simulink model "Ycap_snt"  (R2025b)
settings: Solver=ode45  StartTime=0.0  StopTime=10.0  RelTol=1e-3  EnableMultiTasking=on
undefined symbols (not defined in the file or in its folder): DiscIntNeverNeededParam, Ts
libraries: fl_lib x24, nesl_utility x12
(part 3 of 3)

== system Ycap_snt/3sscT/constPQ2/single-phase PQ/Vectorized PQ meas ==
  V : Inport
  I : Inport  Port=2
  Product1 : Product  InputSameDT=on  SaturateOnIntegerOverflow=on  OutDataTypeStr=Inherit: Same as first input
  Product3 : Product  InputSameDT=on  SaturateOnIntegerOverflow=on  OutDataTypeStr=Inherit: Same as first input
  Sum1 : Sum  Inputs=1  CollapseMode=Specified dimension  InputSameDT=on  SaturateOnIntegerOverflow=on  OutDataTypeStr=Inherit: Same as first input
  Sum2 : Sum  Inputs=1  CollapseMode=Specified dimension  InputSameDT=on  SaturateOnIntegerOverflow=on  OutDataTypeStr=Inherit: Same as first input
  Sum4 : Sum  Inputs=+-  InputSameDT=on  SaturateOnIntegerOverflow=on  OutDataTypeStr=Inherit: Same as first input
  pu->V : Gain  Gain=1/sqrt(3)  SaturateOnIntegerOverflow=on  OutDataTypeStr=Inherit: Same as input  ParamDataTypeStr=Inherit: Same as input
  pu->V1 : Gain  Gain=[0 1 0;0 0 1;1 0 0]  Multiplication=Matrix(K*u)  SaturateOnIntegerOverflow=on  OutDataTypeStr=Inherit: Same as input  ParamDataTypeStr=Inherit: Same as input
  pu->V2 : Gain  Gain=[0 1 0;0 0 1;1 0 0]  Multiplication=Matrix(K*u)  SaturateOnIntegerOverflow=on  OutDataTypeStr=Inherit: Same as input  ParamDataTypeStr=Inherit: Same as input
  P : Outport  VectorParamsAs1DForOutWhenUnconnected=off
  Q : Outport  Port=2  VectorParamsAs1DForOutWhenUnconnected=off
  wires:
  pu->V2/1 -> Product3/1
  Sum4/1 -> pu->V2/1  "VV2"
  pu->V1/1 -> Sum4/2
  Sum2/1 -> P/1
  I/1 -> Product1/2, Product3/2
  V/1 -> Product1/1, pu->V1/1, Sum4/1  "VV1"
  Product1/1 -> Sum2/1
  Product3/1 -> Sum1/1
  Sum1/1 -> pu->V/1
  pu->V/1 -> Q/1

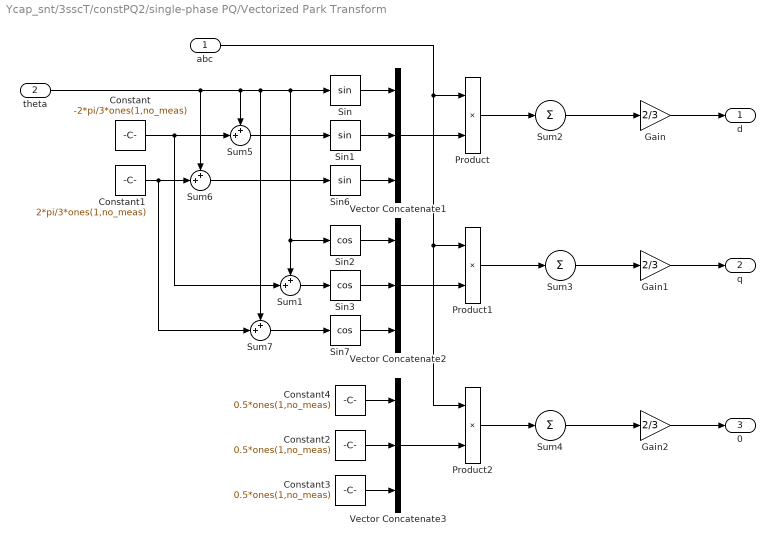
== system Ycap_snt/3sscT/constPQ2/single-phase PQ/Vectorized Park Transform ==
  abc : Inport
  theta : Inport  Port=2
  Constant : Constant  Value=-2*pi/3*ones(1,no_meas)  VectorParams1D=off  SampleTime=Ts
  Constant1 : Constant  Value=2*pi/3*ones(1,no_meas)  VectorParams1D=off  SampleTime=Ts
  Constant2 : Constant  Value=0.5*ones(1,no_meas)  VectorParams1D=off  SampleTime=Ts
  Constant3 : Constant  Value=0.5*ones(1,no_meas)  VectorParams1D=off  SampleTime=Ts
  Constant4 : Constant  Value=0.5*ones(1,no_meas)  VectorParams1D=off  SampleTime=Ts
  Gain : Gain  Gain=2/3
  Gain1 : Gain  Gain=2/3
  Gain2 : Gain  Gain=2/3
  Product : Product
  Product1 : Product
  Product2 : Product
  Sin : Trigonometry
  Sin1 : Trigonometry
  Sin2 : Trigonometry  Operator=cos
  Sin3 : Trigonometry  Operator=cos
  Sin6 : Trigonometry
  Sin7 : Trigonometry  Operator=cos
  Sum{1,5..7} (4 alike) : Sum  Inputs=++|
  Sum2 : Sum  Inputs=1  CollapseMode=Specified dimension  InputSameDT=on  SaturateOnIntegerOverflow=on  OutDataTypeStr=Inherit: Same as first input
  Sum3 : Sum  Inputs=1  CollapseMode=Specified dimension  InputSameDT=on  SaturateOnIntegerOverflow=on  OutDataTypeStr=Inherit: Same as first input
  Sum4 : Sum  Inputs=1  CollapseMode=Specified dimension  InputSameDT=on  SaturateOnIntegerOverflow=on  OutDataTypeStr=Inherit: Same as first input
  Vector Concatenate1 : Concatenate  NumInputs=3  Mode=Multidimensional array
  Vector Concatenate2 : Concatenate  NumInputs=3  Mode=Multidimensional array
  Vector Concatenate3 : Concatenate  NumInputs=3  Mode=Multidimensional array
  d : Outport  VectorParamsAs1DForOutWhenUnconnected=off
  q : Outport  Port=2  VectorParamsAs1DForOutWhenUnconnected=off
  0 : Outport  Port=3  VectorParamsAs1DForOutWhenUnconnected=off
  wires:
  theta/1 -> Sum7/1, Sin/1, Sum1/1, Sin2/1, Sum5/1, Sum6/1
  Sum7/1 -> Sin7/1
  Sum1/1 -> Sin3/1
  Constant1/1 -> Sum6/2, Sum7/2
  Constant/1 -> Sum5/2, Sum1/2
  Sum6/1 -> Sin6/1
  Sum5/1 -> Sin1/1
  abc/1 -> Product2/1, Product1/1, Product/1
  Sin/1 -> Vector Concatenate1/1
  Sin1/1 -> Vector Concatenate1/2
  Sin3/1 -> Vector Concatenate2/2
  Sin2/1 -> Vector Concatenate2/1
  Constant4/1 -> Vector Concatenate3/1
  Constant2/1 -> Vector Concatenate3/2
  Sin6/1 -> Vector Concatenate1/3
  Sin7/1 -> Vector Concatenate2/3
  Constant3/1 -> Vector Concatenate3/3
  Vector Concatenate3/1 -> Product2/2
  Vector Concatenate2/1 -> Product1/2
  Vector Concatenate1/1 -> Product/2
  Product/1 -> Sum2/1
  Product1/1 -> Sum3/1
  Product2/1 -> Sum4/1
  Sum3/1 -> Gain1/1
  Sum4/1 -> Gain2/1
  Sum2/1 -> Gain/1
  Gain2/1 -> 0/1
  Gain1/1 -> q/1
  Gain/1 -> d/1

== system Ycap_snt/3sscT/constPQ2/single-phase PQ/Vectorized Inverse Clarke Transform ==
  alphabeta0 : Inport
  Constant1 : Constant  Value=zeros(1,no_meas)  VectorParams1D=off  SampleTime=Ts
  Constant2 : Constant  Value=sqrt(3)/2*ones(1,no_meas)  VectorParams1D=off  SampleTime=Ts
  Constant3 : Constant  Value=sqrt(1/2)*ones(1,no_meas)  VectorParams1D=off  SampleTime=Ts
  Constant4 : Constant  Value=-0.5*ones(1,no_meas)  VectorParams1D=off  SampleTime=Ts
  Constant5 : Constant  Value=sqrt(1/2)*ones(1,no_meas)  VectorParams1D=off  SampleTime=Ts
  Constant6 : Constant  Value=ones(1,no_meas)  VectorParams1D=off  SampleTime=Ts
  Constant7 : Constant  Value=-sqrt(3)/2*ones(1,no_meas)  VectorParams1D=off  SampleTime=Ts
  Constant8 : Constant  Value=sqrt(1/2)*ones(1,no_meas)  VectorParams1D=off  SampleTime=Ts
  Constant9 : Constant  Value=-0.5*ones(1,no_meas)  VectorParams1D=off  SampleTime=Ts
  Gain : Gain  Gain=sqrt(2/3)
  Gain1 : Gain  Gain=sqrt(2/3)
  Gain2 : Gain  Gain=sqrt(2/3)
  Product : Product
  Product1 : Product
  Product2 : Product
  Sum2 : Sum  Inputs=1  CollapseMode=Specified dimension  InputSameDT=on  SaturateOnIntegerOverflow=on  OutDataTypeStr=Inherit: Same as first input
  Sum3 : Sum  Inputs=1  CollapseMode=Specified dimension  InputSameDT=on  SaturateOnIntegerOverflow=on  OutDataTypeStr=Inherit: Same as first input
  Sum4 : Sum  Inputs=1  CollapseMode=Specified dimension  InputSameDT=on  SaturateOnIntegerOverflow=on  OutDataTypeStr=Inherit: Same as first input
  Vector Concatenate1 : Concatenate  NumInputs=3  Mode=Multidimensional array
  Vector Concatenate2 : Concatenate  NumInputs=3  Mode=Multidimensional array
  Vector Concatenate3 : Concatenate  NumInputs=3  Mode=Multidimensional array
  a : Outport  VectorParamsAs1DForOutWhenUnconnected=off
  b : Outport  Port=2  VectorParamsAs1DForOutWhenUnconnected=off
  c : Outport  Port=3  VectorParamsAs1DForOutWhenUnconnected=off
  wires:
  Constant8/1 -> Vector Concatenate3/3
  Constant7/1 -> Vector Concatenate3/2
  Constant9/1 -> Vector Concatenate3/1
  alphabeta0/1 -> Product/1, Product1/1, Product2/1
  Gain2/1 -> c/1
  Gain1/1 -> b/1
  Gain/1 -> a/1
  Product2/1 -> Sum4/1
  Product1/1 -> Sum3/1
  Product/1 -> Sum2/1
  Vector Concatenate1/1 -> Product/2
  Vector Concatenate2/1 -> Product1/2
  Vector Concatenate3/1 -> Product2/2
  Constant3/1 -> Vector Concatenate2/3
  Constant5/1 -> Vector Concatenate1/3
  Constant4/1 -> Vector Concatenate2/1
  Constant2/1 -> Vector Concatenate2/2
  Constant1/1 -> Vector Concatenate1/2
  Constant6/1 -> Vector Concatenate1/1
  Sum2/1 -> Gain/1
  Sum3/1 -> Gain1/1
  Sum4/1 -> Gain2/1

== system Ycap_snt/3sscT/constPQ2/single-phase PQ/Vectorized Inverse Park Transform ==
  dq0 : Inport
  theta : Inport  Port=2
  Constant : Constant  Value=-2*pi/3*ones(1,no_meas)  VectorParams1D=off  SampleTime=Ts
  Constant1 : Constant  Value=2*pi/3*ones(1,no_meas)  VectorParams1D=off  SampleTime=Ts
  Constant2 : Constant  Value=ones(1,no_meas)  VectorParams1D=off  SampleTime=Ts
  Constant3 : Constant  Value=ones(1,no_meas)  VectorParams1D=off  SampleTime=Ts
  Constant4 : Constant  Value=ones(1,no_meas)  VectorParams1D=off  SampleTime=Ts
  Product : Product
  Product1 : Product
  Product2 : Product
  Sin : Trigonometry
  Sin1 : Trigonometry  Operator=cos
  Sin2 : Trigonometry
  Sin3 : Trigonometry  Operator=cos
  Sin4 : Trigonometry
  Sin5 : Trigonometry  Operator=cos
  Sum : Sum  Inputs=++|
  Sum1 : Sum  Inputs=++|
  Sum2 : Sum  Inputs=1  CollapseMode=Specified dimension  InputSameDT=on  SaturateOnIntegerOverflow=on  OutDataTypeStr=Inherit: Same as first input
  Sum3 : Sum  Inputs=1  CollapseMode=Specified dimension  InputSameDT=on  SaturateOnIntegerOverflow=on  OutDataTypeStr=Inherit: Same as first input
  Sum4 : Sum  Inputs=1  CollapseMode=Specified dimension  InputSameDT=on  SaturateOnIntegerOverflow=on  OutDataTypeStr=Inherit: Same as first input
  Vector Concatenate1 : Concatenate  NumInputs=3  Mode=Multidimensional array
  Vector Concatenate2 : Concatenate  NumInputs=3  Mode=Multidimensional array
  Vector Concatenate3 : Concatenate  NumInputs=3  Mode=Multidimensional array
  a : Outport  VectorParamsAs1DForOutWhenUnconnected=off
  b : Outport  Port=2  VectorParamsAs1DForOutWhenUnconnected=off
  c : Outport  Port=3  VectorParamsAs1DForOutWhenUnconnected=off
  wires:
  Product2/1 -> Sum4/1
  Product1/1 -> Sum3/1
  Product/1 -> Sum2/1
  Vector Concatenate1/1 -> Product/2
  Vector Concatenate2/1 -> Product1/2
  Vector Concatenate3/1 -> Product2/2
  Constant3/1 -> Vector Concatenate3/3
  Constant4/1 -> Vector Concatenate2/3
  Constant2/1 -> Vector Concatenate1/3
  Sin5/1 -> Vector Concatenate3/2
  Sin4/1 -> Vector Concatenate3/1
  Sum1/1 -> Sin5/1, Sin4/1
  Constant1/1 -> Sum1/1
  Constant/1 -> Sum/1
  Sum/1 -> Sin2/1, Sin3/1
  Sin2/1 -> Vector Concatenate2/1
  Sin3/1 -> Vector Concatenate2/2
  Sin1/1 -> Vector Concatenate1/2
  Sin/1 -> Vector Concatenate1/1
  dq0/1 -> Product/1, Product1/1, Product2/1
  theta/1 -> Sum/2, Sin/1, Sum1/2, Sin1/1
  Sum2/1 -> a/1
  Sum3/1 -> b/1
  Sum4/1 -> c/1

== system Ycap_snt/3sscT/constPQ3/single-phase PQ/Subsystem ==
  In1 : Inport
  Discrete-Time Integrator : DiscreteIntegrator  gainval=1/Ts/20  InitialCondition=2000  SampleTime=-1  ICPrevOutput=DiscIntNeverNeededParam  ICPrevScaledInput=DiscIntNeverNeededParam
  Sum : Sum  Inputs=|+-
  Out1 : Outport
  wires:
  In1/1 -> Sum/1
  Sum/1 -> Discrete-Time Integrator/1
  Discrete-Time Integrator/1 -> Sum/2, Out1/1

== system Ycap_snt/3sscT/constPQ3/single-phase PQ/Vectorized Clarke Transform ==
  abc : Inport
  Constant1 : Constant  Value=-0.5*ones(1,no_meas)  VectorParams1D=off  SampleTime=Ts
  Constant{2..4,6} (4 alike) : Constant  Value=ones(1,no_meas)  VectorParams1D=off  SampleTime=Ts
  Constant5 : Constant  Value=-0.5*ones(1,no_meas)  VectorParams1D=off  SampleTime=Ts
  Constant7 : Constant  Value=zeros(1,no_meas)  VectorParams1D=off  SampleTime=Ts
  Constant8 : Constant  Value=sqrt(3)/2*ones(1,no_meas)  VectorParams1D=off  SampleTime=Ts
  Constant9 : Constant  Value=-sqrt(3)/2*ones(1,no_meas)  VectorParams1D=off  SampleTime=Ts
  Gain : Gain  Gain=sqrt(2/3)
  Gain1 : Gain  Gain=sqrt(2/3)
  Gain2 : Gain  Gain=sqrt(1/3)
  Product : Product
  Product1 : Product
  Product2 : Product
  Sum2 : Sum  Inputs=1  CollapseMode=Specified dimension  InputSameDT=on  SaturateOnIntegerOverflow=on  OutDataTypeStr=Inherit: Same as first input
  Sum3 : Sum  Inputs=1  CollapseMode=Specified dimension  InputSameDT=on  SaturateOnIntegerOverflow=on  OutDataTypeStr=Inherit: Same as first input
  Sum4 : Sum  Inputs=1  CollapseMode=Specified dimension  InputSameDT=on  SaturateOnIntegerOverflow=on  OutDataTypeStr=Inherit: Same as first input
  Vector Concatenate1 : Concatenate  NumInputs=3  Mode=Multidimensional array
  Vector Concatenate2 : Concatenate  NumInputs=3  Mode=Multidimensional array
  Vector Concatenate3 : Concatenate  NumInputs=3  Mode=Multidimensional array
  alpha : Outport  VectorParamsAs1DForOutWhenUnconnected=off
  beta : Outport  Port=2  VectorParamsAs1DForOutWhenUnconnected=off
  zero : Outport  Port=3  VectorParamsAs1DForOutWhenUnconnected=off
  wires:
  Gain/1 -> alpha/1
  Gain1/1 -> beta/1
  Gain2/1 -> zero/1
  Sum2/1 -> Gain/1
  Sum4/1 -> Gain2/1
  Sum3/1 -> Gain1/1
  Product2/1 -> Sum4/1
  Product1/1 -> Sum3/1
  Product/1 -> Sum2/1
  Vector Concatenate1/1 -> Product/2
  Vector Concatenate2/1 -> Product1/2
  Vector Concatenate3/1 -> Product2/2
  Constant3/1 -> Vector Concatenate3/3
  Constant2/1 -> Vector Concatenate3/2
  Constant4/1 -> Vector Concatenate3/1
  abc/1 -> Product/1, Product1/1, Product2/1
  Constant6/1 -> Vector Concatenate1/1
  Constant1/1 -> Vector Concatenate1/2
  Constant5/1 -> Vector Concatenate1/3
  Constant7/1 -> Vector Concatenate2/1
  Constant8/1 -> Vector Concatenate2/2
  Constant9/1 -> Vector Concatenate2/3

== system Ycap_snt/3sscT/constPQ3/single-phase PQ/Vectorized PQ meas ==
  V : Inport
  I : Inport  Port=2
  Product1 : Product  InputSameDT=on  SaturateOnIntegerOverflow=on  OutDataTypeStr=Inherit: Same as first input
  Product3 : Product  InputSameDT=on  SaturateOnIntegerOverflow=on  OutDataTypeStr=Inherit: Same as first input
  Sum1 : Sum  Inputs=1  CollapseMode=Specified dimension  InputSameDT=on  SaturateOnIntegerOverflow=on  OutDataTypeStr=Inherit: Same as first input
  Sum2 : Sum  Inputs=1  CollapseMode=Specified dimension  InputSameDT=on  SaturateOnIntegerOverflow=on  OutDataTypeStr=Inherit: Same as first input
  Sum4 : Sum  Inputs=+-  InputSameDT=on  SaturateOnIntegerOverflow=on  OutDataTypeStr=Inherit: Same as first input
  pu->V : Gain  Gain=1/sqrt(3)  SaturateOnIntegerOverflow=on  OutDataTypeStr=Inherit: Same as input  ParamDataTypeStr=Inherit: Same as input
  pu->V1 : Gain  Gain=[0 1 0;0 0 1;1 0 0]  Multiplication=Matrix(K*u)  SaturateOnIntegerOverflow=on  OutDataTypeStr=Inherit: Same as input  ParamDataTypeStr=Inherit: Same as input
  pu->V2 : Gain  Gain=[0 1 0;0 0 1;1 0 0]  Multiplication=Matrix(K*u)  SaturateOnIntegerOverflow=on  OutDataTypeStr=Inherit: Same as input  ParamDataTypeStr=Inherit: Same as input
  P : Outport  VectorParamsAs1DForOutWhenUnconnected=off
  Q : Outport  Port=2  VectorParamsAs1DForOutWhenUnconnected=off
  wires:
  pu->V/1 -> Q/1
  Sum1/1 -> pu->V/1
  Product3/1 -> Sum1/1
  Product1/1 -> Sum2/1
  V/1 -> Sum4/1, pu->V1/1, Product1/1  "VV1"
  I/1 -> Product3/2, Product1/2
  Sum2/1 -> P/1
  pu->V1/1 -> Sum4/2
  Sum4/1 -> pu->V2/1  "VV2"
  pu->V2/1 -> Product3/1

== system Ycap_snt/3sscT/constPQ3/single-phase PQ/Vectorized Park Transform ==
  abc : Inport
  theta : Inport  Port=2
  Constant : Constant  Value=-2*pi/3*ones(1,no_meas)  VectorParams1D=off  SampleTime=Ts
  Constant1 : Constant  Value=2*pi/3*ones(1,no_meas)  VectorParams1D=off  SampleTime=Ts
  Constant2 : Constant  Value=0.5*ones(1,no_meas)  VectorParams1D=off  SampleTime=Ts
  Constant3 : Constant  Value=0.5*ones(1,no_meas)  VectorParams1D=off  SampleTime=Ts
  Constant4 : Constant  Value=0.5*ones(1,no_meas)  VectorParams1D=off  SampleTime=Ts
  Gain : Gain  Gain=2/3
  Gain1 : Gain  Gain=2/3
  Gain2 : Gain  Gain=2/3
  Product : Product
  Product1 : Product
  Product2 : Product
  Sin : Trigonometry
  Sin1 : Trigonometry
  Sin2 : Trigonometry  Operator=cos
  Sin3 : Trigonometry  Operator=cos
  Sin6 : Trigonometry
  Sin7 : Trigonometry  Operator=cos
  Sum{1,5..7} (4 alike) : Sum  Inputs=++|
  Sum2 : Sum  Inputs=1  CollapseMode=Specified dimension  InputSameDT=on  SaturateOnIntegerOverflow=on  OutDataTypeStr=Inherit: Same as first input
  Sum3 : Sum  Inputs=1  CollapseMode=Specified dimension  InputSameDT=on  SaturateOnIntegerOverflow=on  OutDataTypeStr=Inherit: Same as first input
  Sum4 : Sum  Inputs=1  CollapseMode=Specified dimension  InputSameDT=on  SaturateOnIntegerOverflow=on  OutDataTypeStr=Inherit: Same as first input
  Vector Concatenate1 : Concatenate  NumInputs=3  Mode=Multidimensional array
  Vector Concatenate2 : Concatenate  NumInputs=3  Mode=Multidimensional array
  Vector Concatenate3 : Concatenate  NumInputs=3  Mode=Multidimensional array
  d : Outport  VectorParamsAs1DForOutWhenUnconnected=off
  q : Outport  Port=2  VectorParamsAs1DForOutWhenUnconnected=off
  0 : Outport  Port=3  VectorParamsAs1DForOutWhenUnconnected=off
  wires:
  Gain/1 -> d/1
  Gain1/1 -> q/1
  Gain2/1 -> 0/1
  Sum2/1 -> Gain/1
  Sum4/1 -> Gain2/1
  Sum3/1 -> Gain1/1
  Product2/1 -> Sum4/1
  Product1/1 -> Sum3/1
  Product/1 -> Sum2/1
  Vector Concatenate1/1 -> Product/2
  Vector Concatenate2/1 -> Product1/2
  Vector Concatenate3/1 -> Product2/2
  Constant3/1 -> Vector Concatenate3/3
  Sin7/1 -> Vector Concatenate2/3
  Sin6/1 -> Vector Concatenate1/3
  Constant2/1 -> Vector Concatenate3/2
  Constant4/1 -> Vector Concatenate3/1
  Sin2/1 -> Vector Concatenate2/1
  Sin3/1 -> Vector Concatenate2/2
  Sin1/1 -> Vector Concatenate1/2
  Sin/1 -> Vector Concatenate1/1
  abc/1 -> Product/1, Product1/1, Product2/1
  Sum5/1 -> Sin1/1
  Sum6/1 -> Sin6/1
  Constant/1 -> Sum1/2, Sum5/2
  Constant1/1 -> Sum7/2, Sum6/2
  Sum1/1 -> Sin3/1
  Sum7/1 -> Sin7/1
  theta/1 -> Sum6/1, Sum5/1, Sin2/1, Sum1/1, Sin/1, Sum7/1

== system Ycap_snt/3sscT/constPQ3/single-phase PQ/Vectorized Inverse Clarke Transform ==
  alphabeta0 : Inport
  Constant1 : Constant  Value=zeros(1,no_meas)  VectorParams1D=off  SampleTime=Ts
  Constant2 : Constant  Value=sqrt(3)/2*ones(1,no_meas)  VectorParams1D=off  SampleTime=Ts
  Constant3 : Constant  Value=sqrt(1/2)*ones(1,no_meas)  VectorParams1D=off  SampleTime=Ts
  Constant4 : Constant  Value=-0.5*ones(1,no_meas)  VectorParams1D=off  SampleTime=Ts
  Constant5 : Constant  Value=sqrt(1/2)*ones(1,no_meas)  VectorParams1D=off  SampleTime=Ts
  Constant6 : Constant  Value=ones(1,no_meas)  VectorParams1D=off  SampleTime=Ts
  Constant7 : Constant  Value=-sqrt(3)/2*ones(1,no_meas)  VectorParams1D=off  SampleTime=Ts
  Constant8 : Constant  Value=sqrt(1/2)*ones(1,no_meas)  VectorParams1D=off  SampleTime=Ts
  Constant9 : Constant  Value=-0.5*ones(1,no_meas)  VectorParams1D=off  SampleTime=Ts
  Gain : Gain  Gain=sqrt(2/3)
  Gain1 : Gain  Gain=sqrt(2/3)
  Gain2 : Gain  Gain=sqrt(2/3)
  Product : Product
  Product1 : Product
  Product2 : Product
  Sum2 : Sum  Inputs=1  CollapseMode=Specified dimension  InputSameDT=on  SaturateOnIntegerOverflow=on  OutDataTypeStr=Inherit: Same as first input
  Sum3 : Sum  Inputs=1  CollapseMode=Specified dimension  InputSameDT=on  SaturateOnIntegerOverflow=on  OutDataTypeStr=Inherit: Same as first input
  Sum4 : Sum  Inputs=1  CollapseMode=Specified dimension  InputSameDT=on  SaturateOnIntegerOverflow=on  OutDataTypeStr=Inherit: Same as first input
  Vector Concatenate1 : Concatenate  NumInputs=3  Mode=Multidimensional array
  Vector Concatenate2 : Concatenate  NumInputs=3  Mode=Multidimensional array
  Vector Concatenate3 : Concatenate  NumInputs=3  Mode=Multidimensional array
  a : Outport  VectorParamsAs1DForOutWhenUnconnected=off
  b : Outport  Port=2  VectorParamsAs1DForOutWhenUnconnected=off
  c : Outport  Port=3  VectorParamsAs1DForOutWhenUnconnected=off
  wires:
  Sum4/1 -> Gain2/1
  Sum3/1 -> Gain1/1
  Sum2/1 -> Gain/1
  Constant6/1 -> Vector Concatenate1/1
  Constant1/1 -> Vector Concatenate1/2
  Constant2/1 -> Vector Concatenate2/2
  Constant4/1 -> Vector Concatenate2/1
  Constant5/1 -> Vector Concatenate1/3
  Constant3/1 -> Vector Concatenate2/3
  Vector Concatenate3/1 -> Product2/2
  Vector Concatenate2/1 -> Product1/2
  Vector Concatenate1/1 -> Product/2
  Product/1 -> Sum2/1
  Product1/1 -> Sum3/1
  Product2/1 -> Sum4/1
  Gain/1 -> a/1
  Gain1/1 -> b/1
  Gain2/1 -> c/1
  alphabeta0/1 -> Product2/1, Product1/1, Product/1
  Constant9/1 -> Vector Concatenate3/1
  Constant7/1 -> Vector Concatenate3/2
  Constant8/1 -> Vector Concatenate3/3

== system Ycap_snt/3sscT/constPQ3/single-phase PQ/Vectorized Inverse Park Transform ==
  dq0 : Inport
  theta : Inport  Port=2
  Constant : Constant  Value=-2*pi/3*ones(1,no_meas)  VectorParams1D=off  SampleTime=Ts
  Constant1 : Constant  Value=2*pi/3*ones(1,no_meas)  VectorParams1D=off  SampleTime=Ts
  Constant2 : Constant  Value=ones(1,no_meas)  VectorParams1D=off  SampleTime=Ts
  Constant3 : Constant  Value=ones(1,no_meas)  VectorParams1D=off  SampleTime=Ts
  Constant4 : Constant  Value=ones(1,no_meas)  VectorParams1D=off  SampleTime=Ts
  Product : Product
  Product1 : Product
  Product2 : Product
  Sin : Trigonometry
  Sin1 : Trigonometry  Operator=cos
  Sin2 : Trigonometry
  Sin3 : Trigonometry  Operator=cos
  Sin4 : Trigonometry
  Sin5 : Trigonometry  Operator=cos
  Sum : Sum  Inputs=++|
  Sum1 : Sum  Inputs=++|
  Sum2 : Sum  Inputs=1  CollapseMode=Specified dimension  InputSameDT=on  SaturateOnIntegerOverflow=on  OutDataTypeStr=Inherit: Same as first input
  Sum3 : Sum  Inputs=1  CollapseMode=Specified dimension  InputSameDT=on  SaturateOnIntegerOverflow=on  OutDataTypeStr=Inherit: Same as first input
  Sum4 : Sum  Inputs=1  CollapseMode=Specified dimension  InputSameDT=on  SaturateOnIntegerOverflow=on  OutDataTypeStr=Inherit: Same as first input
  Vector Concatenate1 : Concatenate  NumInputs=3  Mode=Multidimensional array
  Vector Concatenate2 : Concatenate  NumInputs=3  Mode=Multidimensional array
  Vector Concatenate3 : Concatenate  NumInputs=3  Mode=Multidimensional array
  a : Outport  VectorParamsAs1DForOutWhenUnconnected=off
  b : Outport  Port=2  VectorParamsAs1DForOutWhenUnconnected=off
  c : Outport  Port=3  VectorParamsAs1DForOutWhenUnconnected=off
  wires:
  Sum4/1 -> c/1
  Sum3/1 -> b/1
  Sum2/1 -> a/1
  theta/1 -> Sin1/1, Sum1/2, Sin/1, Sum/2
  dq0/1 -> Product2/1, Product1/1, Product/1
  Sin/1 -> Vector Concatenate1/1
  Sin1/1 -> Vector Concatenate1/2
  Sin3/1 -> Vector Concatenate2/2
  Sin2/1 -> Vector Concatenate2/1
  Sum/1 -> Sin3/1, Sin2/1
  Constant/1 -> Sum/1
  Constant1/1 -> Sum1/1
  Sum1/1 -> Sin4/1, Sin5/1
  Sin4/1 -> Vector Concatenate3/1
  Sin5/1 -> Vector Concatenate3/2
  Constant2/1 -> Vector Concatenate1/3
  Constant4/1 -> Vector Concatenate2/3
  Constant3/1 -> Vector Concatenate3/3
  Vector Concatenate3/1 -> Product2/2
  Vector Concatenate2/1 -> Product1/2
  Vector Concatenate1/1 -> Product/2
  Product/1 -> Sum2/1
  Product1/1 -> Sum3/1
  Product2/1 -> Sum4/1
